simulink model "serial_i2c_PCF8474Read"  (R2016b)
settings: Solver=FixedStepDiscrete  StartTime=0.0  StopTime=10.0  FixedStep=1e-3  RelTol=1e-3
libraries: mbed_lib x6, simulink x3
settings Model: Creator=oh  LastModifiedBy=oh
settings DataIOCC: LimitDataPoints=on  SaveFormat=Array
settings OptimizationCC: LifeSpan=1
settings DebuggingCC: SFUnexpectedBacktrackingDiag=warning  SFNoUnconditionalDefaultTransitionDiag=warning  SFExecutionAtInitializationDiag=none
settings HardwareCC: ProdBitPerPointer=32  ProdBitPerSizeT=32  ProdBitPerPtrDiffT=32  ProdLargestAtomicInteger=Long  ProdLargestAtomicFloat=Double  ProdIntDivRoundTo=Undefined  ProdWordSize=32  ProdHWDeviceType=ARM Compatible->ARM Cortex
settings ModelReferenceCC: PropagateSignalLabelsOutOfModel=off
settings RTWCC: SystemTargetFile=mbed.tlc  TemplateMakefile=mbed.tmf  Description=Mbed Target (Embedded Target)  TargetLang=C++
settings CodeAppCC: IgnoreCustomStorageClasses=off
settings STFCustomTargetCC: TargetLibSuffix=.a  GenerateSampleERTMain=on  CombineOutputUpdateFcns=on  ERTCustomFileBanners=on  SupportContinuousTime=off  SupportNonInlinedSFcns=off  RemoveResetFunc=on  MATLABClassNameForMDSCustomization=Simulink.SoftwareTarget.ERTCustomization  GRTInterface=off  SystemTargetFile=mbed.tlc
settings ERTTargetCC: GenerateSampleERTMain=on  ParMdlRefBuildCompliant=off  CompOptLevelCompliant=off  ConcurrentExecutionCompliant=off  ERTFirstTimeCompliant=off  ModelStepFunctionPrototypeControlCompliant=off  CPPClassGenCompliant=off  UseToolchainInfoCompliant=off  ERTCustomFileTemplate=mbed_file_process.tlc  ConvertIfToSwitch=off  SuppressUnreachableDefaultCases=off
settings ConfigComp: CovMetricSettings=dw  CovHtmlReporting=on  CovSaveCumulativeToWorkspaceVar=on  CovSaveSingleToWorkspaceVar=on  CovExternalEMLEnable=off

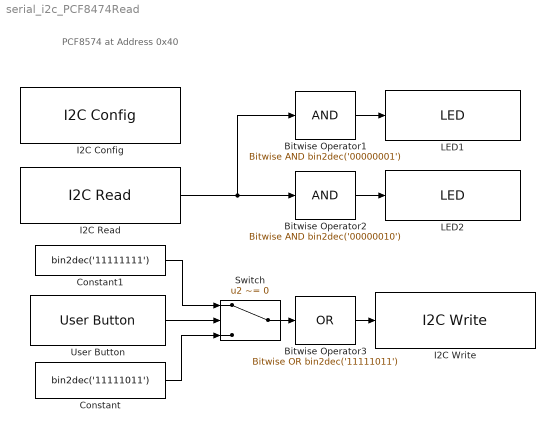
== system serial_i2c_PCF8474Read ==
  note: PCF8574 at Address 0x40
  Bitwise Operator1 : simulink/Logic and Bit Operations/Bitwise Operator  logicop=AND  UseBitMask=on  BitMask=bin2dec('00000001')  BitMaskRealWorld=Stored Integer
  Bitwise Operator2 : simulink/Logic and Bit Operations/Bitwise Operator  logicop=AND  UseBitMask=on  BitMask=bin2dec('00000010')  BitMaskRealWorld=Stored Integer
  Bitwise Operator3 : simulink/Logic and Bit Operations/Bitwise Operator  logicop=OR  UseBitMask=on  BitMask=bin2dec('11111011')  BitMaskRealWorld=Stored Integer
  Constant : Constant  Value=bin2dec('11111011')  OutDataTypeStr=uint8
  Constant1 : Constant  Value=bin2dec('11111111')  OutDataTypeStr=uint8
  I2C Config : mbed_lib/Serial/I2C/I2C Config  Priority=0  I2CPort=1  Freq=100000  SDAPortName=B  SDAPinNumber=9  SCLPortName=B  SCLPinNumber=8
  I2C Read : mbed_lib/Serial/I2C/I2C Read  I2cPort=1  AddressFlag=off  SlaveAddress=64  ByteCountFlag=off  NumBytes=1  Repeated=off  AckOut=off  SampleTime=0.1
  I2C Write : mbed_lib/Serial/I2C/I2C Write  I2cPort=1  AddressFlag=off  SlaveAddress=64  ByteCountFlag=off  Repeated=off  AckOut=off  SampleTime=-1
  LED1 : mbed_lib/GPIO/LED  nLED=1  SampleTime=-1
  LED2 : mbed_lib/GPIO/LED  nLED=2  SampleTime=-1
  Switch : Switch  Criteria=u2 ~= 0
  User Button : mbed_lib/GPIO/User Button  SampleTime=0.1
  wires:
  Bitwise Operator1/1 -> LED1/1
  Bitwise Operator2/1 -> LED2/1
  Switch/1 -> Bitwise Operator3/1
  User Button/1 -> Switch/2
  Bitwise Operator3/1 -> I2C Write/1
  Constant1/1 -> Switch/1
  Constant/1 -> Switch/3
  I2C Read/1 -> Bitwise Operator1/1, Bitwise Operator2/1
